simulink model "OpenLoop"  (R2024a)
settings: Solver=ode4  StartTime=0.0  StopTime=inf  FixedStep=DT  MaxStep=DT  RelTol=1e-3  EnableMultiTasking=on
values from neighbouring files (symbols this model uses):
  agent = agent.saved_agent    [Run_OpenLoop.m]
  rate = 1    [Run_OpenLoop.m]
  Ts = 0.025    [Run_OpenLoop.m]
undefined symbols (not defined in the file or in its folder): OutList, strmatch
libraries: simulink x2, rllib x1
settings Model: Creator=bjonkman  LastModifiedBy=vicemora
settings SolverCC: AlgebraicLoopSolver=TrustRegion
settings DataIOCC: LimitDataPoints=on  SaveFormat=Array  SignalLoggingSaveFormat=ModelDataLogs  SaveOutput=off  SaveTime=off  SignalLoggingName=sigsOut
settings OptimizationCC: ExpressionDepthLimit=2147483647  LifeSpan=inf
settings DebuggingCC: SaveWithParameterizedLinksMsg=none  UnderspecifiedInitializationDetection=Classic  MergeDetectMultiDrivingBlocksExec=none  SignalResolutionControl=TryResolveAllWithWarning  MultiTaskDSMMsg=warning  MultiTaskCondExecSysMsg=none  FcnCallInpInsideContextMsg=warning  UnconnectedInputMsg=warning  UnconnectedOutputMsg=warning  UnconnectedLineMsg=warning  StateNameClashWarn=warning  SFUnexpectedBacktrackingDiag=warning  SFNoUnconditionalDefaultTransitionDiag=warning  SFExecutionAtInitializationDiag=none  ArithmeticOperatorsInVariantConditions=warning
settings HardwareCC: ProdBitPerPointer=32  ProdBitPerSizeT=32  ProdBitPerPtrDiffT=32  ProdLargestAtomicFloat=None  ProdIntDivRoundTo=Undefined  ProdEndianess=Unspecified  ProdWordSize=32  ProdHWDeviceType=32-bit Generic  TargetUnknown=on
settings ModelReferenceCC: EnableRefExpFcnMdlSchedulingChecks=on  PropagateSignalLabelsOutOfModel=off
settings SFSimCC: SimUseLocalCustomCode=off  CustomCodeUndefinedFunction=UseInterfaceOnly
settings RTWCC: RTWUseLocalCustomCode=off  GPUComputeCapability=3.5  DLArmComputeVersion=19.05
settings CodeAppCC: StateflowObjectComments=on
settings GRTTargetCC: TargetLangStandard=C89/C90 (ANSI)  CombineOutputUpdateFcns=off  GRTInterface=on
settings ConfigComp: CovMetricSettings=dw  CovSaveCumulativeToWorkspaceVar=on  CovSaveSingleToWorkspaceVar=on  CovExternalEMLEnable=off

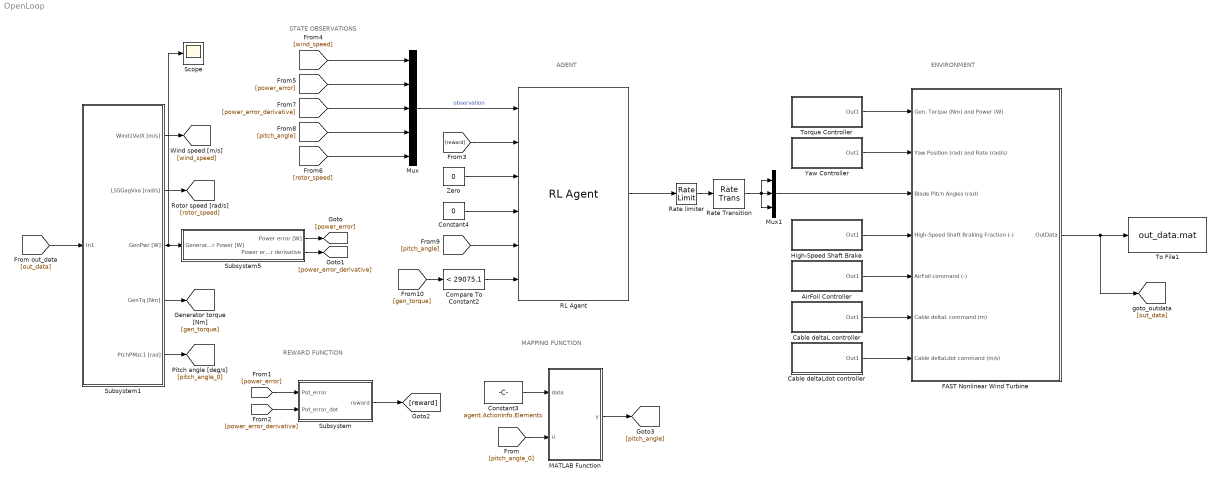
== system OpenLoop ==
  note: STATE OBSERVATIONS
  note: REWARD FUNCTION
  note: AGENT
  note: ENVIRONMENT
  note: MAPPING FUNCTION
  AirFoil Controller : Subsystem
  Cable deltaL controller : Subsystem
  Cable deltaLdot controller : Subsystem
  Compare To Constant2 : simulink/Logic and Bit Operations/Compare To Constant  relop=<  const=29075.1  OutDataTypeStr=boolean
  Constant3 : Constant  Value=agent.ActionInfo.Elements
  Constant4 : Constant  Value=0
  FAST Nonlinear Wind Turbine : Subsystem  mask(FAST Nonlinear Wind Turbine){}
      mask help: This block contains the FAST S-Function.
      mask init:
      | clear FAST_SFunc
  High-Speed Shaft Brake : Subsystem
  MATLAB Function : MATLAB Function  TreatAsAtomicUnit=on
  Mux : Mux  Inputs=5
  Mux1 : Mux  Inputs=3
  RL Agent : rllib/RL Agent  Agent=agent  ExternalActionAsInput=on  ProvideLastAction=on  ProvideCumRwd=off  TreatAsDirectFeedthrough=on  UseStrictObservationDataTypes=off
  Rate Transition : RateTransition  OutPortSampleTime=0.025
  Rate limiter : RateLimiter  RisingSlewLimit=rate*pi/180  FallingSlewLimit=-rate*pi/180  SampleTimeMode=inherited  LinearizeAsGain=off
  Scope : Scope
  Subsystem : Subsystem
  Subsystem1 : Subsystem
  Subsystem5 : Subsystem
  To File1 : ToFile  Filename=out_data.mat  MatrixName=data
  Torque Controller : Subsystem
  Yaw Controller : Subsystem
  Zero : Constant  Value=0  OutDataTypeStr=Inherit: Inherit via back propagation
  wires:
  Torque Controller/1(Out1) -> FAST Nonlinear Wind Turbine/1(Gen. Torque (Nm) and Power (W))
  Yaw Controller/1(Out1) -> FAST Nonlinear Wind Turbine/2(Yaw Position (rad) and Rate (rad/s))
  High-Speed Shaft Brake/1(Out1) -> FAST Nonlinear Wind Turbine/4(High-Speed Shaft Braking Fraction (-))
  AirFoil Controller/1(Out1) -> FAST Nonlinear Wind Turbine/5(AirFoil command (-))
  Cable deltaL controller/1(Out1) -> FAST Nonlinear Wind Turbine/6(Cable deltaL command (m))
  Cable deltaLdot controller/1(Out1) -> FAST Nonlinear Wind Turbine/7(Cable deltaLdot command (m/s))
  Mux/1 -> RL Agent/1  "observation"
  Zero/1 -> RL Agent/3
  Mux1/1 -> FAST Nonlinear Wind Turbine/3(Blade Pitch Angles (rad))
  Constant3/1 -> MATLAB Function/1(data)
  FAST Nonlinear Wind Turbine/1(OutData) -> To File1/1, [out_data]
  [out_data] -> Subsystem1/1(In1)
  Rate limiter/1 -> Rate Transition/1
  RL Agent/1 -> Rate limiter/1
  Rate Transition/1 -> Mux1/1, Mux1/3, Mux1/2
  Compare To Constant2/1 -> RL Agent/6
  Subsystem1/3(GenPwr [W]) -> Scope/1, Subsystem5/1(Generator Power [W])
  Subsystem1/4(GenTq [Nm]) -> [gen_torque]
  Subsystem1/1(Wind1VelX [m/s]) -> [wind_speed]
  Subsystem1/2(LSSGagVxa [rad/s]) -> [rotor_speed]
  Subsystem1/5(PtchPMzc1 [rad]) -> [pitch_angle_0]
  [pitch_angle_0] -> MATLAB Function/2(u)
  Subsystem5/2(Power error derivative) -> [power_error_derivative]
  Subsystem5/1(Power error [W]) -> [power_error]
  [power_error] -> Subsystem/1(Pot_error)
  [power_error_derivative] -> Subsystem/2(Pot_error_dot)
  Subsystem/1(reward) -> [reward]
  [reward] -> RL Agent/2
  [wind_speed] -> Mux/1
  [power_error] -> Mux/2
  [power_error_derivative] -> Mux/3
  [rotor_speed] -> Mux/5
  MATLAB Function/1(y) -> [pitch_angle]
  [pitch_angle] -> Mux/4
  [pitch_angle] -> RL Agent/5
  Constant4/1 -> RL Agent/4
  [gen_torque] -> Compare To Constant2/1

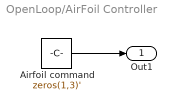
== system OpenLoop/AirFoil Controller ==
  Airfoil command : Constant  Value=zeros(1,3)'
  Out1 : Outport
  wires:
  Airfoil command/1 -> Out1/1

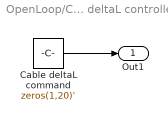
== system OpenLoop/Cable deltaL controller ==
  Cable deltaL command : Constant  Value=zeros(1,20)'
  Out1 : Outport
  wires:
  Cable deltaL command/1 -> Out1/1

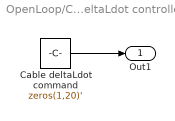
== system OpenLoop/Cable deltaLdot controller ==
  Cable deltaLdot command : Constant  Value=zeros(1,20)'
  Out1 : Outport
  wires:
  Cable deltaLdot command/1 -> Out1/1

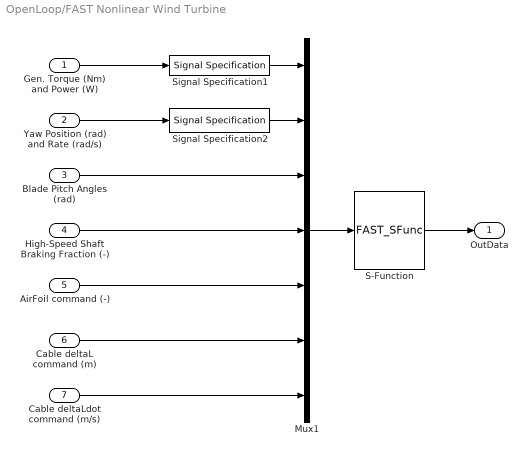
== system OpenLoop/FAST Nonlinear Wind Turbine ==
  Gen. Torque (Nm) and Power (W) : Inport
  Yaw Position (rad) and Rate (rad/s) : Inport  Port=2
  Blade Pitch Angles (rad) : Inport  Port=3
  High-Speed Shaft Braking Fraction (-) : Inport  Port=4
  AirFoil command (-) : Inport  Port=5
  Cable deltaL command (m) : Inport  Port=6
  Cable deltaLdot command (m/s) : Inport  Port=7
  Mux1 : Mux  Inputs=7
  S-Function : S-Function  FunctionName=FAST_SFunc  Parameters=FAST_InputFileName, TMax, 0  SFunctionDeploymentMode=off  EnableBusSupport=off
  Signal Specification1 : SignalSpecification  OutDataTypeStr=double  Dimensions=2
  Signal Specification2 : SignalSpecification  OutDataTypeStr=double  Dimensions=2
  OutData : Outport
  wires:
  Gen. Torque (Nm) and Power (W)/1 -> Signal Specification1/1
  S-Function/1 -> OutData/1
  Mux1/1 -> S-Function/1
  Blade Pitch Angles (rad)/1 -> Mux1/3
  Yaw Position (rad) and Rate (rad/s)/1 -> Signal Specification2/1
  Signal Specification1/1 -> Mux1/1
  Signal Specification2/1 -> Mux1/2
  High-Speed Shaft Braking Fraction (-)/1 -> Mux1/4
  AirFoil command (-)/1 -> Mux1/5
  Cable deltaL command (m)/1 -> Mux1/6
  Cable deltaLdot command (m/s)/1 -> Mux1/7

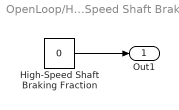
== system OpenLoop/High-Speed Shaft Brake ==
  High-Speed Shaft Braking Fraction : Constant  Value=0
  Out1 : Outport
  wires:
  High-Speed Shaft Braking Fraction/1 -> Out1/1

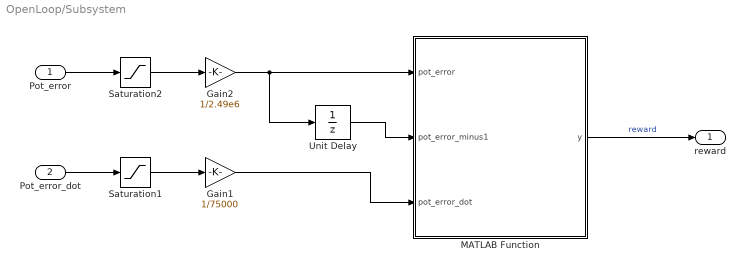
== system OpenLoop/Subsystem ==
  Pot_error : Inport
  Pot_error_dot : Inport  Port=2
  Gain1 : Gain  Gain=1/75000
  Gain2 : Gain  Gain=1/2.49e6
  MATLAB Function : MATLAB Function  TreatAsAtomicUnit=on
  Saturation1 : Saturate  UpperLimit=75000  LowerLimit=-75000
  Saturation2 : Saturate  UpperLimit=2.49e6  LowerLimit=-2.49e6
  Unit Delay : UnitDelay  SampleTime=Ts  HasFrameUpgradeWarning=on
  reward : Outport
  wires:
  MATLAB Function/1(y) -> reward/1  "reward"
  Pot_error/1 -> Saturation2/1
  Unit Delay/1 -> MATLAB Function/2(pot_error_minus1)
  Pot_error_dot/1 -> Saturation1/1
  Gain2/1 -> Unit Delay/1, MATLAB Function/1(pot_error)
  Gain1/1 -> MATLAB Function/3(pot_error_dot)
  Saturation2/1 -> Gain2/1
  Saturation1/1 -> Gain1/1

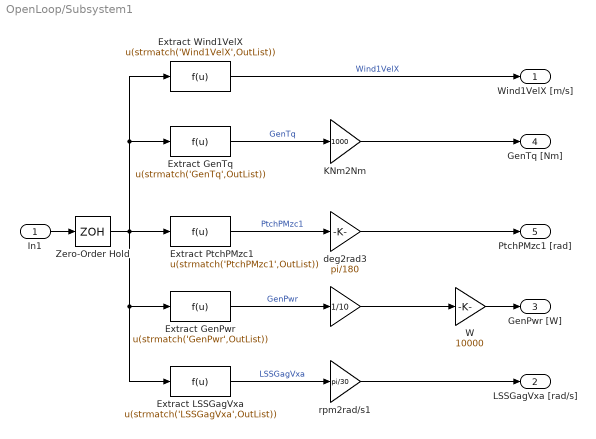
== system OpenLoop/Subsystem1 ==
  In1 : Inport
  " " : Gain  Gain=1/10
  Extract GenPwr : Fcn  Expr=u(strmatch('GenPwr',OutList))
  Extract GenTq : Fcn  Expr=u(strmatch('GenTq',OutList))
  Extract LSSGagVxa : Fcn  Expr=u(strmatch('LSSGagVxa',OutList))
  Extract PtchPMzc1 : Fcn  Expr=u(strmatch('PtchPMzc1',OutList))
  Extract Wind1VelX : Fcn  Expr=u(strmatch('Wind1VelX',OutList))
  KNm2Nm : Gain  Gain=1000
  W : Gain  Gain=10000
  Zero-Order Hold : ZeroOrderHold  SampleTime=Ts
  deg2rad3 : Gain  Gain=pi/180
  rpm2rad/s1 : Gain  Gain=pi/30
  Wind1VelX [m/s] : Outport
  LSSGagVxa [rad/s] : Outport  Port=2
  GenPwr [W] : Outport  Port=3
  GenTq [Nm] : Outport  Port=4
  PtchPMzc1 [rad] : Outport  Port=5
  wires:
  KNm2Nm/1 -> GenTq [Nm]/1
  Extract GenTq/1 -> KNm2Nm/1  "GenTq"
  Extract Wind1VelX/1 -> Wind1VelX [m/s]/1  "Wind1VelX"
  deg2rad3/1 -> PtchPMzc1 [rad]/1
  Extract PtchPMzc1/1 -> deg2rad3/1  "PtchPMzc1"
  Extract LSSGagVxa/1 -> rpm2rad/s1/1  "LSSGagVxa"
  Extract GenPwr/1 -> " "/1  "GenPwr"
  rpm2rad/s1/1 -> LSSGagVxa [rad/s]/1
  W/1 -> GenPwr [W]/1
  " "/1 -> W/1
  In1/1 -> Zero-Order Hold/1
  Zero-Order Hold/1 -> Extract LSSGagVxa/1, Extract GenPwr/1, Extract GenTq/1, Extract Wind1VelX/1, Extract PtchPMzc1/1

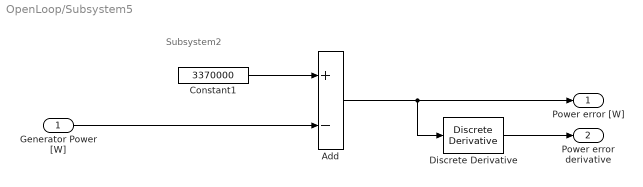
== system OpenLoop/Subsystem5 ==
  note: Subsystem2
  Generator Power [W] : Inport
  Add : Sum  Inputs=+-
  Constant1 : Constant  Value=3370000  SampleTime=Ts
  Discrete Derivative : simulink/Discrete/Discrete Derivative  gainval=1.0  ICPrevScaledInput=0.0  OutMin=[]  OutMax=[]  OutDataType=fixdt(1, 16)  OutScaling=2^-10  DoSatur=off
  Power error [W] : Outport
  Power error derivative : Outport  Port=2
  wires:
  Discrete Derivative/1 -> Power error derivative/1
  Add/1 -> Discrete Derivative/1, Power error [W]/1
  Generator Power [W]/1 -> Add/2
  Constant1/1 -> Add/1

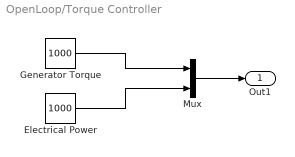
== system OpenLoop/Torque Controller ==
  Electrical Power : Constant  Value=1000
  Generator Torque : Constant  Value=1000
  Mux : Mux  Inputs=2
  Out1 : Outport
  wires:
  Mux/1 -> Out1/1
  Generator Torque/1 -> Mux/1
  Electrical Power/1 -> Mux/2

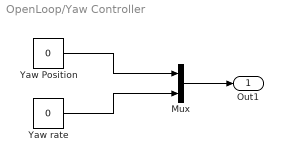
== system OpenLoop/Yaw Controller ==
  Mux : Mux  Inputs=2
  Yaw Position : Constant  Value=0
  Yaw rate : Constant  Value=0
  Out1 : Outport
  wires:
  Mux/1 -> Out1/1
  Yaw Position/1 -> Mux/1
  Yaw rate/1 -> Mux/2

== matlab function OpenLoop/MATLAB Function ==
  data: data input; u input; y output
function y = fcn(data, u)
if u>data(1) && u<data(end)
    y=data(discretize(u,data));
else
    if u<=data(1)
        y=data(1);
    else
        y=data(end);
    end
end

== matlab function OpenLoop/Subsystem/MATLAB Function ==
  data: y output; pot_error input; pot_error_minus1 input; pot_error_dot input
function y = fcn(pot_error, pot_error_minus1, pot_error_dot)
if (pot_error>0 && pot_error_dot>0) || (pot_error<0 && pot_error_dot<0)
    rv=-abs(pot_error_dot);
elseif (pot_error>0 && pot_error_dot<0) || (pot_error<0 && pot_error_dot>0)
    if abs(pot_error_dot)>0.3
        rv=abs(pot_error_dot)*abs(pot_error);
    else 
        rv=abs(pot_error_dot)*2*(1-abs(pot_error));
    end
else
    rv=-abs(pot_error_dot);
end

if sign(pot_error)~=sign(pot_error_minus1) && abs(pot_error)<abs(pot_error_minus1)
    rt=-rv;
else
    rt=rv;
end

y=rt-abs(pot_error);
